simulink model "obiekt_regulator"  (R2016b)
settings: Solver=VariableStepAuto  StartTime=0.0  StopTime=5.0  RelTol=1e-3
values from neighbouring files (symbols this model uses):
  A1 = A.'    [z1.m]
  B1 = C.'    [z1.m]
  K = acker(A1,B1,p)    [z1.m]
settings Model: Creator=kamil  LastModifiedBy=kamil

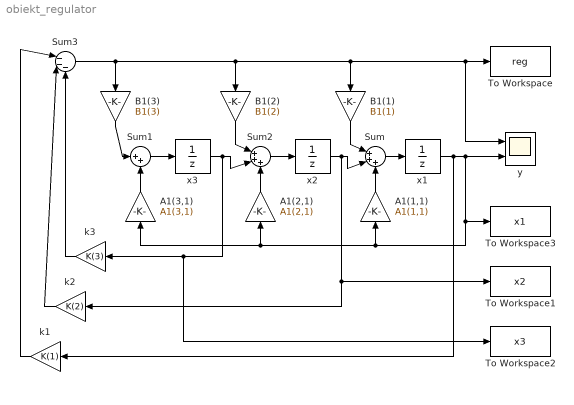
== system obiekt_regulator ==
  A1(1,1) : Gain  Gain=A1(1,1)
  A1(2,1) : Gain  Gain=A1(2,1)
  A1(3,1) : Gain  Gain=A1(3,1)
  B1(1) : Gain  Gain=B1(1)
  B1(2) : Gain  Gain=B1(2)
  B1(3) : Gain  Gain=B1(3)
  Sum : Sum  Inputs=|+++
  Sum1 : Sum  Inputs=|++
  Sum2 : Sum  Inputs=|+++
  Sum3 : Sum  Inputs=|---
  To Workspace : ToWorkspace  VariableName=reg  SaveFormat=Structure With Time  SampleTime=-1
  To Workspace1 : ToWorkspace  VariableName=x2  SaveFormat=Structure With Time  SampleTime=-1
  To Workspace2 : ToWorkspace  VariableName=x3  SaveFormat=Structure With Time  SampleTime=-1
  To Workspace3 : ToWorkspace  VariableName=x1  SaveFormat=Structure With Time  SampleTime=-1
  k1 : Gain  Gain=K(1)
  k2 : Gain  Gain=K(2)
  k3 : Gain  Gain=K(3)
  x1 : UnitDelay  InitialCondition=3  SampleTime=-1
  x2 : UnitDelay  InitialCondition=-1  SampleTime=-1
  x3 : UnitDelay  InitialCondition=1  SampleTime=-1
  y : Scope  NumInputPorts=2
  wires:
  B1(3)/1 -> Sum1/1
  Sum3/1 -> To Workspace/1, y/1, B1(1)/1, B1(2)/1, B1(3)/1
  Sum1/1 -> x3/1
  A1(1,1)/1 -> Sum/3
  A1(2,1)/1 -> Sum2/3
  A1(3,1)/1 -> Sum1/2
  Sum/1 -> x1/1
  x2/1 -> To Workspace1/1, k2/1, Sum/2
  Sum2/1 -> x2/1
  B1(1)/1 -> Sum/1
  B1(2)/1 -> Sum2/1
  k3/1 -> Sum3/3
  k2/1 -> Sum3/2
  k1/1 -> Sum3/1
  x1/1 -> k1/1, y/2, To Workspace3/1, A1(3,1)/1, A1(2,1)/1, A1(1,1)/1
  x3/1 -> To Workspace2/1, k3/1, Sum2/2
